simulink model "integral_control"  (R2016a)
settings: Solver=VariableStepAuto  StartTime=0.0  StopTime=.1  RelTol=1e-4
undefined symbols (not defined in the file): K, K1, K2
settings Model: Creator=manuel  LastModifiedBy=manuel

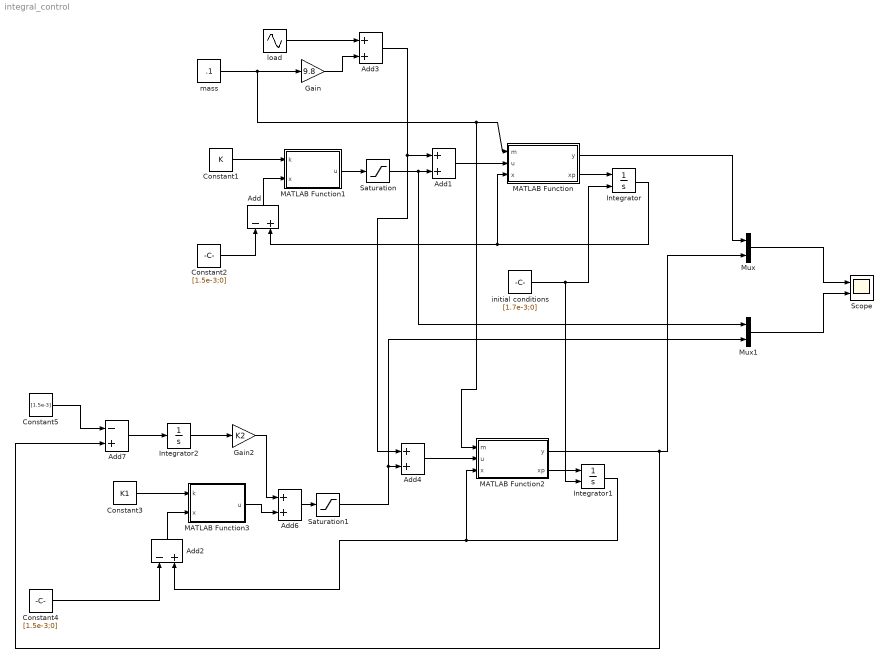
== system integral_control ==
  Add : Sum  Inputs=-+
  Add{1,3..4,6} (4 alike) : Sum
  Add2 : Sum  Inputs=-+
  Add7 : Sum  Inputs=-+
  Constant1 : Constant  Value=K
  Constant2 : Constant  Value=[1.5e-3;0]
  Constant3 : Constant  Value=K1
  Constant4 : Constant  Value=[1.5e-3;0]
  Constant5 : Constant  Value=[1.5e-3]
  Gain : Gain  Gain=9.8
  Gain2 : Gain  Gain=K2
  Integrator : Integrator  InitialConditionSource=external  InitialCondition=[1.6e-3;0]  LimitOutput=on  UpperSaturationLimit=[2e-3;inf]  LowerSaturationLimit=[1e-3;-inf]
  Integrator1 : Integrator  InitialConditionSource=external  InitialCondition=[1.6e-3;0]  LimitOutput=on  UpperSaturationLimit=[2e-3;inf]  LowerSaturationLimit=[1e-3;-inf]
  Integrator2 : Integrator  InitialCondition=[0]  UpperSaturationLimit=[2e-3;inf]  LowerSaturationLimit=[1e-3;-inf]
  MATLAB Function : MATLAB Function  TreatAsAtomicUnit=on
  MATLAB Function1 : MATLAB Function  TreatAsAtomicUnit=on
  MATLAB Function2 : MATLAB Function  TreatAsAtomicUnit=on
  MATLAB Function3 : MATLAB Function  TreatAsAtomicUnit=on
  Mux : Mux  Inputs=2
  Mux1 : Mux  Inputs=2
  Saturation : Saturate  UpperLimit=9.8  LowerLimit=-9.8
  Saturation1 : Saturate  UpperLimit=9.8  LowerLimit=-9.8
  Scope : Scope  NumInputPorts=2
  initial conditions : Constant  Value=[1.7e-3;0]
  load : Sin  Bias=1  Frequency=2*pi*100  SampleTime=0
  mass : Constant  Value=.1
  wires:
  MATLAB Function/2(xp) -> Integrator/1
  Integrator/1 -> MATLAB Function/3(x), Add/2
  MATLAB Function/1(y) -> Mux/1
  Constant1/1 -> MATLAB Function1/1(k)
  Constant2/1 -> Add/1
  Add/1 -> MATLAB Function1/2(x)
  Add1/1 -> MATLAB Function/2(u)
  Gain/1 -> Add3/2
  load/1 -> Add3/1
  Mux/1 -> Scope/1
  Mux1/1 -> Scope/2
  MATLAB Function1/1(u) -> Saturation/1
  Saturation/1 -> Mux1/1, Add1/2
  MATLAB Function2/2(xp) -> Integrator1/1
  Integrator1/1 -> Add2/2, MATLAB Function2/3(x)
  MATLAB Function2/1(y) -> Add7/2, Mux/2
  Constant3/1 -> MATLAB Function3/1(k)
  Constant4/1 -> Add2/1
  Add2/1 -> MATLAB Function3/2(x)
  Add4/1 -> MATLAB Function2/2(u)
  Add3/1 -> Add4/1, Add1/1
  initial conditions/1 -> Integrator1/2, Integrator/2
  Saturation1/1 -> Mux1/2, Add4/2
  Integrator2/1 -> Gain2/1
  Add6/1 -> Saturation1/1
  Gain2/1 -> Add6/1
  MATLAB Function3/1(u) -> Add6/2
  Add7/1 -> Integrator2/1
  Constant5/1 -> Add7/1
  mass/1 -> Gain/1, MATLAB Function2/1(m), MATLAB Function/1(m)

== matlab function integral_control/MATLAB Function1 ==
  data: k input; x input; u output
function u = fcn(k,x)
%#codegen

u = -k'*x;

== matlab function integral_control/MATLAB Function ==
  data: m input; u input; x input; y output; xp output
function [y,xp] = mass_model(m,u,x)
%#codegen
A = [0 1
     0 0];
B = [0;
     1/m];
C = [1 0];

xp = A*x + B*u;
y = C*x;

== matlab function integral_control/MATLAB Function2 ==
  data: m input; u input; x input; y output; xp output
function [y,xp] = mass_model(m,u,x)
%#codegen
A = [0 1
     0 0];
B = [0;
     1/m];
C = [1 0];

xp = A*x + B*u;
y = C*x;

== matlab function integral_control/MATLAB Function3 ==
  data: k input; x input; u output
function u = fcn(k,x)
%#codegen

u = -k'*x;
